simulink model "SegheriaSCADA"  (R2024b)
settings: Solver=FixedStepAuto  StartTime=0.0  StopTime=100  FixedStep=0.01  MaxStep=0.01  RelTol=1e-3
values from neighbouring files (symbols this model uses):
  b = t + 2*s    (= 3.6)    [ParametriSegheria.m]    (also in ParametriSegheriaDinamica.m)
  b2 = t2 + 2*s2    (= 10)    [ParametriSegheria.m]    (also in ParametriSegheriaDinamica.m)
  h1 = 70    [ParametriSegheria.m]
  h2 = 18    [ParametriSegheria.m]
  i_id = 60    [ParametriSegheria.m]
  i_id2 = 60    [ParametriSegheria.m]
  kc = [0 35 40 50 55 90]    [ParametriSegheria.m]    (also in ParametriSegheriaDinamica.m = [0, 25, 30, 35, 50, 70])
  Kt = 2    [ParametriSegheria.m]    (also in ParametriSegheriaDinamica.m = 10000)
  Kt2 = 5    [ParametriSegheria.m]    (also in ParametriSegheriaDinamica.m = 4500)
  Lt = 4    [ParametriSegheria.m]    (also in ParametriSegheriaDinamica.m)
  Mag_D = [0 430 320 260 230 540]    [ParametriSegheria.m]    (also in ParametriSegheriaDinamica.m = [0 randi([220 500], 1, 150)])
  Mag_legno = [0 1 5 2 4 3]    [ParametriSegheria.m]    (also in ParametriSegheriaDinamica.m = [0 randi([1 5], 1, 150)])
  n_sottili = 4    [ParametriSegheria.m]    (also in ParametriSegheriaDinamica.m)
  omega = 50    [ParametriSegheria.m]
  omega2 = 3000*(2*pi/60)    (= 314.159265359)    [ParametriSegheria.m]
  SR = Rs/Rm    (= 5.33333333333)    [ParametriSegheria.m]    (also in ParametriSegheriaDinamica.m)
  SR2 = Rc/Rm2    (= 4)    [ParametriSegheria.m]    (also in ParametriSegheriaDinamica.m)
  Tloss = Tatt+ Tdamp    (= 17.3333333333)    [ParametriSegheria.m]
  Tloss2 = Tatt2+ Tdamp2    (= 66.8318530718)    [ParametriSegheria.m]
  w = 50    [ParametriSegheria.m]
undefined symbols (not defined in the file or in its folder): i_max
libraries: simulink x3, slpidlib x2
settings Model: Creator=samue  LastModifiedBy=samue

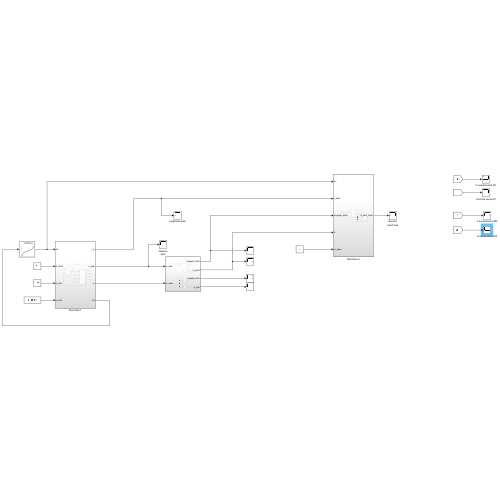
[thumbnail: Simulink's stored preview of the top-level diagram]
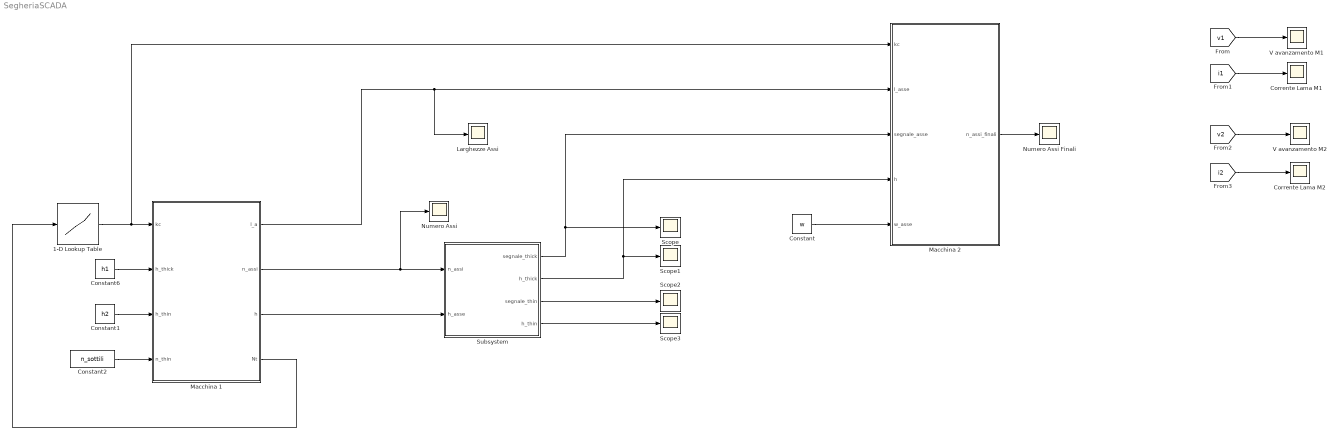
== system SegheriaSCADA ==
  1-D Lookup Table : Lookup_n-D  NumberOfTableDimensions=1  BreakpointsForDimension1=[0 1 2 3 4 5 ]  Table=kc  InternalRulePriority=Speed  RndMeth=Simplest
  Constant : Constant  Value=w
  Constant1 : Constant  Value=h2
  Constant2 : Constant  Value=n_sottili
  Constant6 : Constant  Value=h1
  Corrente Lama M1 : Scope
  Corrente Lama M2 : Scope
  Larghezze Assi : Scope
  Macchina 1 : Subsystem
  Macchina 2 : Subsystem
  Numero Assi : Scope
  Numero Assi Finali : Scope
  Scope{,1..3} (4 alike) : Scope
  Subsystem : Subsystem
  V avanzamento M1 : Scope
  V avanzamento M2 : Scope
  wires:
  Macchina 1/4(Nt) -> 1-D Lookup Table/1
  1-D Lookup Table/1 -> Macchina 2/1(kc), Macchina 1/1(kc)
  Macchina 1/2(n_assi) -> Numero Assi/1, Subsystem/1(n_assi)
  Macchina 1/1(l_a) -> Macchina 2/2(l_asse), Larghezze Assi/1
  Macchina 2/1(n_assi_finali) -> Numero Assi Finali/1
  Constant/1 -> Macchina 2/5(w_asse)
  Constant6/1 -> Macchina 1/2(h_thick)
  [i2] -> Corrente Lama M2/1
  [v2] -> V avanzamento M2/1
  [v1] -> V avanzamento M1/1
  [i1] -> Corrente Lama M1/1
  Constant1/1 -> Macchina 1/3(h_thin)
  Constant2/1 -> Macchina 1/4(n_thin)
  Macchina 1/3(h) -> Subsystem/2(h_asse)
  Subsystem/1(segnale_thick) -> Macchina 2/3(segnale_asse), Scope/1
  Subsystem/2(h_thick) -> Scope1/1, Macchina 2/4(h)
  Subsystem/3(segnale_thin) -> Scope2/1
  Subsystem/4(h_thin) -> Scope3/1

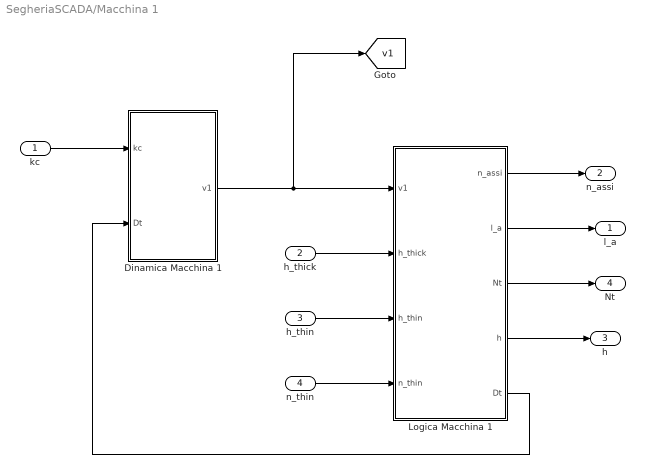
== system SegheriaSCADA/Macchina 1 ==
  kc : Inport
  h_thick : Inport  Port=2
  h_thin : Inport  Port=3
  n_thin : Inport  Port=4
  Dinamica Macchina 1 : Subsystem
  Logica Macchina 1 : Subsystem
  l_a : Outport
  n_assi : Outport  Port=2
  h : Outport  Port=3
  Nt : Outport  Port=4
  tag scope: v1=global
  wires:
  kc/1 -> Dinamica Macchina 1/1(kc)
  Dinamica Macchina 1/1(v1) -> [v1], Logica Macchina 1/1(v1)
  Logica Macchina 1/3(Nt) -> Nt/1
  Logica Macchina 1/5(Dt) -> Dinamica Macchina 1/2(Dt)
  Logica Macchina 1/1(n_assi) -> n_assi/1
  Logica Macchina 1/2(l_a) -> l_a/1
  h_thick/1 -> Logica Macchina 1/2(h_thick)
  h_thin/1 -> Logica Macchina 1/3(h_thin)
  n_thin/1 -> Logica Macchina 1/4(n_thin)
  Logica Macchina 1/4(h) -> h/1

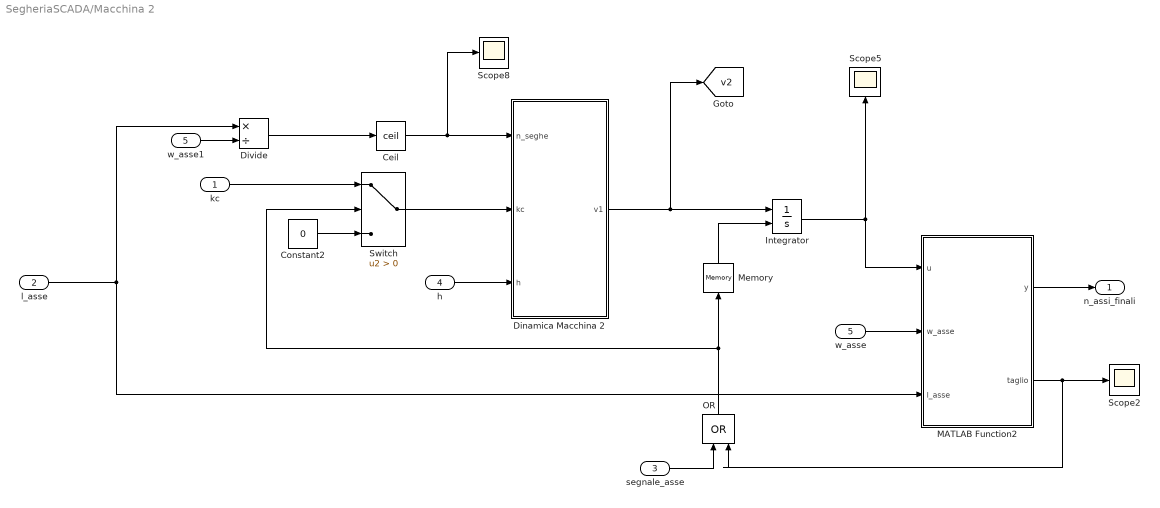
== system SegheriaSCADA/Macchina 2 ==
  kc : Inport
  l_asse : Inport  Port=2
  segnale_asse : Inport  Port=3
  h : Inport  Port=4
  w_asse : Inport  Port=5
  Ceil : Rounding  Operator=ceil
  Constant2 : Constant  Value=0
  Dinamica Macchina 2 : Subsystem
  Divide : Product  Inputs=*/
  Integrator : Integrator  ExternalReset=falling
  MATLAB Function2 : MATLAB Function  TreatAsAtomicUnit=on
  Memory : Memory
  OR : Logic  Operator=OR  IconShape=distinctive  AllPortsSameDT=off  OutDataTypeStr=boolean
  Scope2 : Scope
  Scope5 : Scope
  Scope8 : Scope
  Switch : Switch  Criteria=u2 > Threshold  SaturateOnIntegerOverflow=off  InputSameDT=off
  w_asse1 : InportShadow  Port=5
  n_assi_finali : Outport
  tag scope: v2=global
  wires:
  Divide/1 -> Ceil/1
  OR/1 -> Switch/2, Memory/1
  Dinamica Macchina 2/1(v1) -> [v2], Integrator/1
  Constant2/1 -> Switch/3
  Switch/1 -> Dinamica Macchina 2/2(kc)
  Integrator/1 -> Scope5/1, MATLAB Function2/1(u)
  w_asse/1 -> MATLAB Function2/2(w_asse)
  MATLAB Function2/2(taglio) -> Scope2/1, OR/2
  h/1 -> Dinamica Macchina 2/3(h)
  l_asse/1 -> MATLAB Function2/3(l_asse), Divide/1
  Ceil/1 -> Scope8/1, Dinamica Macchina 2/1(n_seghe)
  Memory/1 -> Integrator/2
  kc/1 -> Switch/1
  MATLAB Function2/1(y) -> n_assi_finali/1
  w_asse1/1 -> Divide/2
  segnale_asse/1 -> OR/1

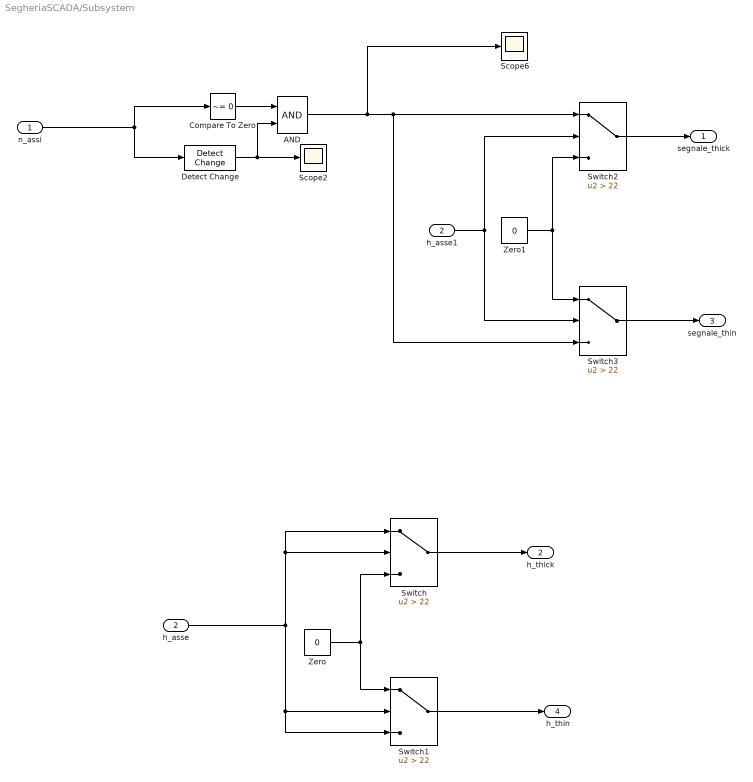
== system SegheriaSCADA/Subsystem ==
  n_assi : Inport
  h_asse : Inport  Port=2
  AND : Logic  IconShape=distinctive  AllPortsSameDT=off  OutDataTypeStr=boolean
  Compare To Zero : simulink/Logic and Bit Operations/Compare To Zero  relop=~=  OutDataTypeStr=boolean
  Detect Change : simulink/Logic and Bit Operations/Detect Change  vinit=0  OutDataTypeStr=boolean
  Scope2 : Scope
  Scope6 : Scope
  Switch{,1..3} (4 alike) : Switch  Criteria=u2 > Threshold  Threshold=22  SaturateOnIntegerOverflow=off  InputSameDT=off
  Zero : Constant  Value=0  OutDataTypeStr=Inherit: Inherit via back propagation
  Zero1 : Constant  Value=0  OutDataTypeStr=Inherit: Inherit via back propagation
  h_asse1 : InportShadow  Port=2
  segnale_thick : Outport
  h_thick : Outport  Port=2
  segnale_thin : Outport  Port=3
  h_thin : Outport  Port=4
  wires:
  Detect Change/1 -> Scope2/1, AND/2
  Zero/1 -> Switch1/1, Switch/3
  Switch/1 -> h_thick/1
  n_assi/1 -> Compare To Zero/1, Detect Change/1
  Compare To Zero/1 -> AND/1
  Switch1/1 -> h_thin/1
  Zero1/1 -> Switch2/3, Switch3/1
  h_asse/1 -> Switch/1, Switch/2, Switch1/2, Switch1/3
  Switch2/1 -> segnale_thick/1
  h_asse1/1 -> Switch2/2, Switch3/2
  AND/1 -> Switch3/3, Switch2/1, Scope6/1
  Switch3/1 -> segnale_thin/1

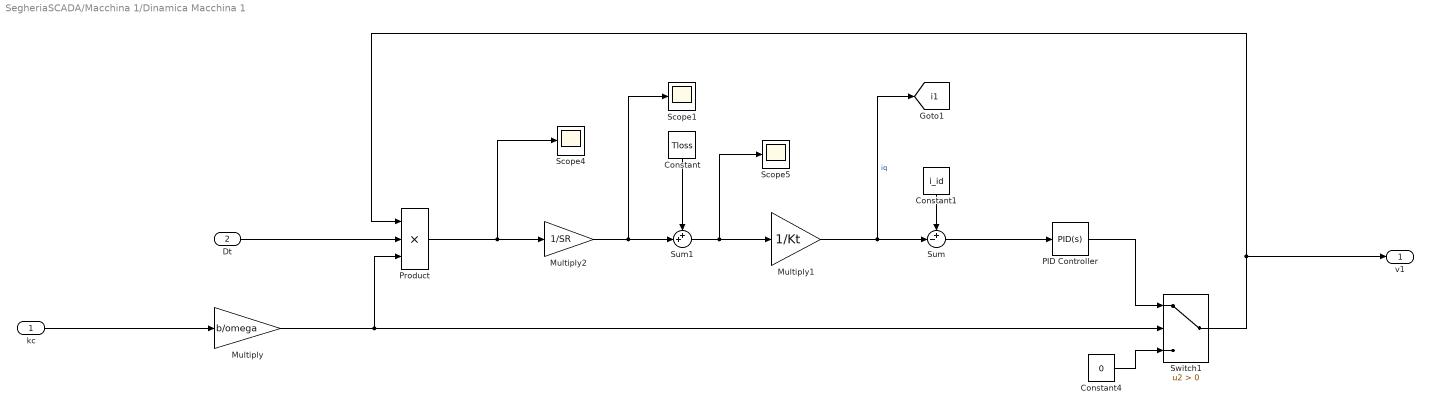
== system SegheriaSCADA/Macchina 1/Dinamica Macchina 1 ==
  kc : Inport
  Dt : Inport  Port=2
  Constant : Constant  Value=Tloss
  Constant1 : Constant  Value=i_id
  Constant4 : Constant  Value=0
  Multiply : Gain  Gain=b/omega
  Multiply1 : Gain  Gain=1/Kt
  Multiply2 : Gain  Gain=1/SR
  PID Controller : slpidlib/PID Controller  Controller=PID  Form=Parallel  TimeDomain=Continuous-time  UseExternalTs=off  SampleTime=-1  IntegratorMethod=Forward Euler  FilterMethod=Forward Euler  ControllerParametersSource=internal  P=0  I=0.0048685791703887  UseKiTs=off  D=0  UseExternalDerivativeSource=off  N=100  UseFilter=on  TunerSelectOption=Transfer Function Based (PID Tuner App)  InitialConditionSource=internal  InitialConditionForIntegrator=0  InitialConditionForFilter=0  DifferentiatorICPrevScaledInput=0  ExternalReset=none  TrackingMode=off  Kt=1  LimitOutput=off  SatLimitsSource=internal  UpperSaturationLimit=i_max  LowerSaturationLimit=-inf  LinearizeAsGain=on  AntiWindupMode=none  Kb=1  LimitIntegrator=off  UpperIntegratorSaturationLimit=inf  LowerIntegratorSaturationLimit=-inf  POutMin=[]  POutMax=[]  IOutMin=[]  IOutMax=[]  DOutMin=[]  DOutMax=[]  NOutMin=[]  NOutMax=[]  SumOutMin=[]  SumOutMax=[]  SaturationOutMin=[]  SaturationOutMax=[]  PParamMin=[]  PParamMax=[]  IParamMin=[]  IParamMax=[]  DParamMin=[]  DParamMax=[]  NParamMin=[]  NParamMax=[]  KbParamMin=[]  KbParamMax=[]  KtParamMin=[]  KtParamMax=[]  KbOutMin=[]  KbOutMax=[]  KtOutMin=[]  KtOutMax=[]  IntegratorOutMin=[]  IntegratorOutMax=[]  FilterOutMin=[]  FilterOutMax=[]  SumI1OutMin=[]  SumI1OutMax=[]  SumI2OutMin=[]  SumI2OutMax=[]  SumI3OutMin=[]  SumI3OutMax=[]  SumI4OutMin=[]  SumI4OutMax=[]  SumDOutMin=[]  SumDOutMax=[]  DifferentiatorOutMin=[]  DifferentiatorOutMax=[]  FilterDiffOutCoefMin=[]  FilterDiffOutCoefMax=[]  ReciprocalOutMin=[]  ReciprocalOutMax=[]  SumDenOutMin=[]  SumDenOutMax=[]  SumNumOutMin=[]  SumNumOutMax=[]  DivideOutMin=[]  DivideOutMax=[]  UdiffTsProdOutMin=[]  UdiffTsProdOutMax=[]  NTsProdOutMin=[]  NTsProdOutMax=[]  UintegralTsProdOutMin=[]  UintegralTsProdOutMax=[]  UngainTsProdOutMin=[]  UngainTsProdOutMax=[]  ClampingZeroOutDataTypeStr=Inherit: Inherit via back propagation  ClampingZeroOutMin=[]  ClampingZeroOutMax=[]  FilterDenConstantOutDataTypeStr=Inherit: Inherit via back propagation  FilterDenConstantOutMin=[]  FilterDenConstantOutMax=[]  PCopyOutDataTypeStr=Inherit: Inherit via back propagation  PCopyOutMin=[]  PCopyOutMax=[]  NCopyOutDataTypeStr=Inherit: Inherit via back propagation  NCopyOutMin=[]  NCopyOutMax=[]  IntegratorContinuousStateAttributes=''  IntegratorStateMustResolveToSignalObject=off  IntegratorRTWStateStorageClass=Auto  FilterContinuousStateAttributes=''  FilterStateMustResolveToSignalObject=off  FilterRTWStateStorageClass=Auto  ParallelPVariant=InternalParameters  IdealPVariant=Disabled  IVariant=InternalParameters  DVariant=InternalParameters  IntegratorVariant=Continuous  SatVariant=Disabled  AWVariant=Passthrough  PCopyVariant=Disabled  TRVariant=Disabled  FdbkBlocksVariant=Forward  IdealPFdbkVariant=Disabled  SatFdbkVariant=Disabled  DerivativeFilterVariant=ContFilter  NVariant=InternalParameters  NCopyVariant=Disabled  FilterICVariant=InternalICsFilter  IntegratorICVariant=InternalICs  ExternalResetVariant=Disabled  TRSumVariant=Passthrough  SumFdbkVariant=Disabled  SumVariant=Sum_PID  TsampFilterVariant=InternalTs  TsampNgainVariant=Passthrough  TsampIntegralVariant=Disabled_SignalSpec  ExternalSaturationOutDataTypeStr=Inherit: Same as second input  DerivativeSourceVariant=ErrorSignal  PreIntVariant=InternalPreInt
  Product : Product  Inputs=3
  Scope1 : Scope
  Scope4 : Scope
  Scope5 : Scope
  Sum : Sum  Inputs=+-|
  Sum1 : Sum  Inputs=++|
  Switch1 : Switch  Criteria=u2 > Threshold  SaturateOnIntegerOverflow=off  InputSameDT=off
  v1 : Outport
  tag scope: i1=global
  wires:
  Constant4/1 -> Switch1/3
  Product/1 -> Scope4/1, Multiply2/1
  PID Controller/1 -> Switch1/1
  Multiply1/1 -> [i1], Sum/2  "iq"
  Multiply/1 -> Product/3, Switch1/2
  kc/1 -> Multiply/1
  Switch1/1 -> v1/1, Product/1
  Constant1/1 -> Sum/1
  Sum/1 -> PID Controller/1
  Multiply2/1 -> Sum1/2, Scope1/1
  Sum1/1 -> Scope5/1, Multiply1/1
  Constant/1 -> Sum1/1
  Dt/1 -> Product/2

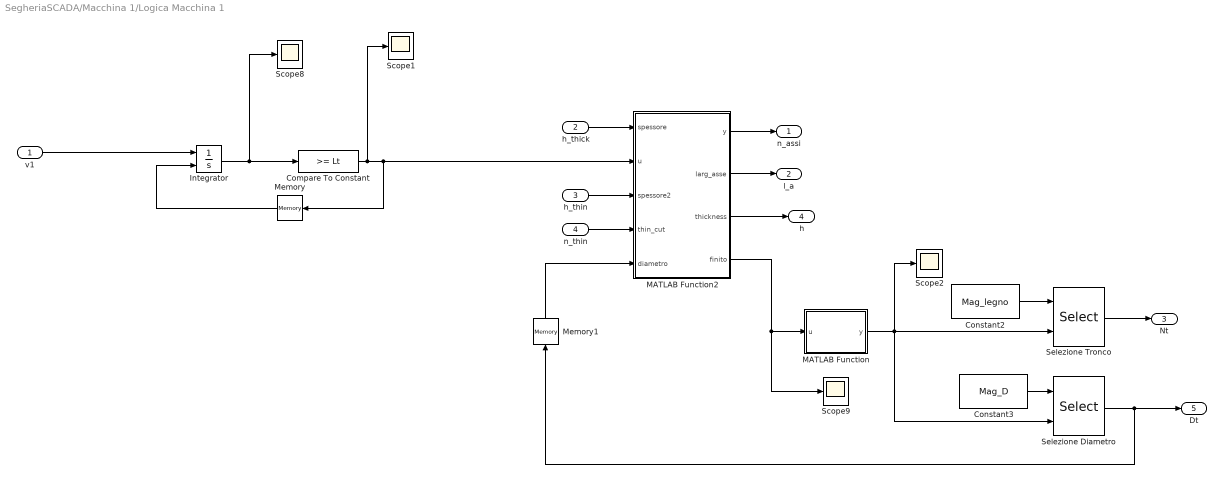
== system SegheriaSCADA/Macchina 1/Logica Macchina 1 ==
  v1 : Inport
  h_thick : Inport  Port=2
  h_thin : Inport  Port=3
  n_thin : Inport  Port=4
  Compare To Constant : simulink/Logic and Bit Operations/Compare To Constant  relop=>=  const=Lt  OutDataTypeStr=boolean
  Constant2 : Constant  Value=Mag_legno
  Constant3 : Constant  Value=Mag_D
  Integrator : Integrator  ExternalReset=rising
  MATLAB Function : MATLAB Function  TreatAsAtomicUnit=on
  MATLAB Function2 : MATLAB Function  TreatAsAtomicUnit=on
  Memory : Memory
  Memory1 : Memory
  Scope{1..2,8..9} (4 alike) : Scope
  Selezione Diametro : Selector  IndexMode=Zero-based  InputPortWidth=length(Mag_D)  IndexOptions=Index vector (port)  Indices=[1 3]  OutputSizes=1
  Selezione Tronco : Selector  IndexMode=Zero-based  InputPortWidth=length(Mag_legno)  IndexOptions=Index vector (port)  Indices=[1 3]  OutputSizes=1
  n_assi : Outport
  l_a : Outport  Port=2
  Nt : Outport  Port=3
  h : Outport  Port=4
  Dt : Outport  Port=5
  wires:
  Selezione Diametro/1 -> Dt/1, Memory1/1
  MATLAB Function2/4(finito) -> MATLAB Function/1(u), Scope9/1
  Memory/1 -> Integrator/2
  Memory1/1 -> MATLAB Function2/5(diametro)
  Constant2/1 -> Selezione Tronco/1
  v1/1 -> Integrator/1
  Integrator/1 -> Compare To Constant/1, Scope8/1
  Constant3/1 -> Selezione Diametro/1
  MATLAB Function/1(y) -> Selezione Diametro/2, Scope2/1, Selezione Tronco/2
  MATLAB Function2/1(y) -> n_assi/1
  Selezione Tronco/1 -> Nt/1
  MATLAB Function2/2(larg_asse) -> l_a/1
  Compare To Constant/1 -> Scope1/1, Memory/1, MATLAB Function2/2(u)
  h_thick/1 -> MATLAB Function2/1(spessore)
  h_thin/1 -> MATLAB Function2/3(spessore2)
  n_thin/1 -> MATLAB Function2/4(thin_cut)
  MATLAB Function2/3(thickness) -> h/1

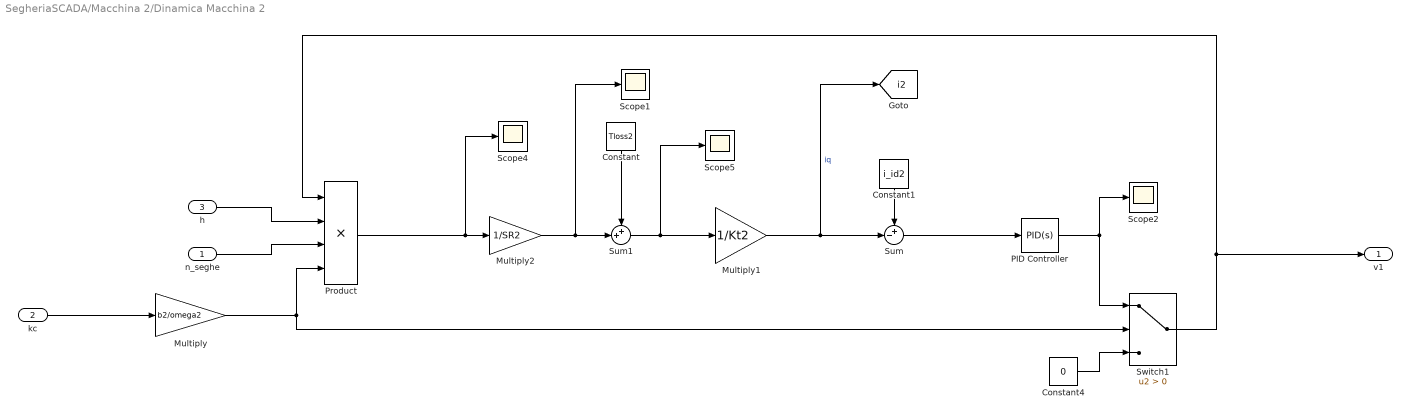
== system SegheriaSCADA/Macchina 2/Dinamica Macchina 2 ==
  n_seghe : Inport
  kc : Inport  Port=2
  h : Inport  Port=3
  Constant : Constant  Value=Tloss2
  Constant1 : Constant  Value=i_id2
  Constant4 : Constant  Value=0
  Multiply : Gain  Gain=b2/omega2
  Multiply1 : Gain  Gain=1/Kt2
  Multiply2 : Gain  Gain=1/SR2
  PID Controller : slpidlib/PID Controller  Controller=PID  Form=Parallel  TimeDomain=Continuous-time  UseExternalTs=off  SampleTime=-1  IntegratorMethod=Forward Euler  FilterMethod=Forward Euler  ControllerParametersSource=internal  P=0.1  I=0  UseKiTs=off  D=0  UseExternalDerivativeSource=off  N=100  UseFilter=on  TunerSelectOption=Transfer Function Based (PID Tuner App)  InitialConditionSource=internal  InitialConditionForIntegrator=0  InitialConditionForFilter=0  DifferentiatorICPrevScaledInput=0  ExternalReset=none  TrackingMode=off  Kt=1  LimitOutput=off  SatLimitsSource=internal  UpperSaturationLimit=1.7  LowerSaturationLimit=0  LinearizeAsGain=on  AntiWindupMode=none  Kb=1  LimitIntegrator=off  UpperIntegratorSaturationLimit=inf  LowerIntegratorSaturationLimit=-inf  POutMin=[]  POutMax=[]  IOutMin=[]  IOutMax=[]  DOutMin=[]  DOutMax=[]  NOutMin=[]  NOutMax=[]  SumOutMin=[]  SumOutMax=[]  SaturationOutMin=[]  SaturationOutMax=[]  PParamMin=[]  PParamMax=[]  IParamMin=[]  IParamMax=[]  DParamMin=[]  DParamMax=[]  NParamMin=[]  NParamMax=[]  KbParamMin=[]  KbParamMax=[]  KtParamMin=[]  KtParamMax=[]  KbOutMin=[]  KbOutMax=[]  KtOutMin=[]  KtOutMax=[]  IntegratorOutMin=[]  IntegratorOutMax=[]  FilterOutMin=[]  FilterOutMax=[]  SumI1OutMin=[]  SumI1OutMax=[]  SumI2OutMin=[]  SumI2OutMax=[]  SumI3OutMin=[]  SumI3OutMax=[]  SumI4OutMin=[]  SumI4OutMax=[]  SumDOutMin=[]  SumDOutMax=[]  DifferentiatorOutMin=[]  DifferentiatorOutMax=[]  FilterDiffOutCoefMin=[]  FilterDiffOutCoefMax=[]  ReciprocalOutMin=[]  ReciprocalOutMax=[]  SumDenOutMin=[]  SumDenOutMax=[]  SumNumOutMin=[]  SumNumOutMax=[]  DivideOutMin=[]  DivideOutMax=[]  UdiffTsProdOutMin=[]  UdiffTsProdOutMax=[]  NTsProdOutMin=[]  NTsProdOutMax=[]  UintegralTsProdOutMin=[]  UintegralTsProdOutMax=[]  UngainTsProdOutMin=[]  UngainTsProdOutMax=[]  ClampingZeroOutDataTypeStr=Inherit: Inherit via back propagation  ClampingZeroOutMin=[]  ClampingZeroOutMax=[]  FilterDenConstantOutDataTypeStr=Inherit: Inherit via back propagation  FilterDenConstantOutMin=[]  FilterDenConstantOutMax=[]  PCopyOutDataTypeStr=Inherit: Inherit via back propagation  PCopyOutMin=[]  PCopyOutMax=[]  NCopyOutDataTypeStr=Inherit: Inherit via back propagation  NCopyOutMin=[]  NCopyOutMax=[]  IntegratorContinuousStateAttributes=''  IntegratorStateMustResolveToSignalObject=off  IntegratorRTWStateStorageClass=Auto  FilterContinuousStateAttributes=''  FilterStateMustResolveToSignalObject=off  FilterRTWStateStorageClass=Auto  ParallelPVariant=InternalParameters  IdealPVariant=Disabled  IVariant=InternalParameters  DVariant=InternalParameters  IntegratorVariant=Continuous  SatVariant=Disabled  AWVariant=Passthrough  PCopyVariant=Disabled  TRVariant=Disabled  FdbkBlocksVariant=Forward  IdealPFdbkVariant=Disabled  SatFdbkVariant=Disabled  DerivativeFilterVariant=ContFilter  NVariant=InternalParameters  NCopyVariant=Disabled  FilterICVariant=InternalICsFilter  IntegratorICVariant=InternalICs  ExternalResetVariant=Disabled  TRSumVariant=Passthrough  SumFdbkVariant=Disabled  SumVariant=Sum_PID  TsampFilterVariant=InternalTs  TsampNgainVariant=Passthrough  TsampIntegralVariant=Disabled_SignalSpec  ExternalSaturationOutDataTypeStr=Inherit: Same as second input  DerivativeSourceVariant=ErrorSignal  PreIntVariant=InternalPreInt
  Product : Product  Inputs=4
  Scope{1..2,4..5} (4 alike) : Scope
  Sum : Sum  Inputs=+-|
  Sum1 : Sum  Inputs=++|
  Switch1 : Switch  Criteria=u2 > Threshold  SaturateOnIntegerOverflow=off  InputSameDT=off
  v1 : Outport
  tag scope: i2=global
  wires:
  Constant4/1 -> Switch1/3
  Product/1 -> Scope4/1, Multiply2/1
  PID Controller/1 -> Switch1/1, Scope2/1
  Multiply1/1 -> [i2], Sum/2  "iq"
  Multiply/1 -> Product/4, Switch1/2
  kc/1 -> Multiply/1
  Switch1/1 -> v1/1, Product/1
  Constant1/1 -> Sum/1
  Sum/1 -> PID Controller/1
  Multiply2/1 -> Scope1/1, Sum1/2
  Sum1/1 -> Scope5/1, Multiply1/1
  Constant/1 -> Sum1/1
  h/1 -> Product/2
  n_seghe/1 -> Product/3

== matlab function SegheriaSCADA/Macchina 2/MATLAB Function2 ==
  settings: updateMethod=DISCRETE
  data: u input; w_asse input; y output; l_asse input; taglio output; Lt parameter
function [y, taglio] = fcn(u, w_asse, l_asse, Lt)
    persistent counter 

    n_assi = floor(l_asse / w_asse);
    
    taglio = 0;

    if isempty(counter)
        counter = 0;
    end

    % Conto assi tagliate
    if u >= Lt
        counter = counter + n_assi;
    end

    % Segnale di taglio
    if  (u > 0 && u < Lt && l_asse > 0) 
        taglio = 1;
    end

    y = counter;
end

== matlab function SegheriaSCADA/Macchina 1/Logica Macchina 1/MATLAB Function ==
  data: u input; y output; Mag_legno parameter
function y = fcn(u, Mag_legno)
    persistent counter
    if isempty(counter)
        counter = 1;
    end

    if u == 1
        counter = counter + 1;
    end

    y = counter;
    
    if y > length(Mag_legno)-1
        y = 0;
    end

end

== matlab function SegheriaSCADA/Macchina 1/Logica Macchina 1/MATLAB Function2 ==
  settings: updateMethod=DISCRETE
  data: spessore input; u input; spessore2 input; thin_cut input; diametro input; y output; larg_asse output; thickness output; finito output
function [y, larg_asse, thickness, finito]= fcn(spessore, u, spessore2, thin_cut, diametro)
    persistent counter 

  
    max_assi = floor((diametro-thin_cut*spessore2) / spessore);
    finito = 0;
    
    if isempty(counter)
        counter = 0;
    end

    % Conto assi tagliate
    if u == 1
        counter = counter + 1;
    end

    % Quando finisco tronco segnalo e azzero counter
    if counter > max_assi + thin_cut
        finito = 1;
        counter = 0;
    end

    
    if counter == 0
        larg_asse = 0;
        thickness = 0;
    elseif counter <= thin_cut/2
        distanza_bordo = counter * spessore2;
        h = abs(diametro/2 - distanza_bordo + (spessore2/2));
        larg_asse = 2 * sqrt((diametro/2)^2-h^2);
        thickness = spessore2;
    elseif counter > max_assi + thin_cut/2
        distanza_bordo = max_assi*spessore + (counter-max_assi)*spessore2;
        h = abs(diametro/2 - distanza_bordo + (spessore2/2));
        larg_asse = 2 * sqrt((diametro/2)^2-h^2);
        thickness = spessore2;
    else
        % Calcolo larghezza delle assi
        distanza_bordo = thin_cut/2 * spessore2 + (counter-thin_cut/2) * spessore;
        h = abs(diametro/2 - distanza_bordo + (spessore/2));
        larg_asse = 2 * sqrt((diametro/2)^2-h^2);
        thickness = spessore;
    end
    

    y = counter;
